simulink model "filter_2nd_order_iir_cosim"  (Simulink 6.4)
settings: Solver=FixedStepDiscrete  SolverMode=SingleTasking  StartTime=0.0  StopTime=0.1  RelTol=1e-3
undefined symbols (not defined in the file or in its folder): pipeline_prec
libraries: modelsimlib x1
settings Model: LastModifiedBy=Administrador

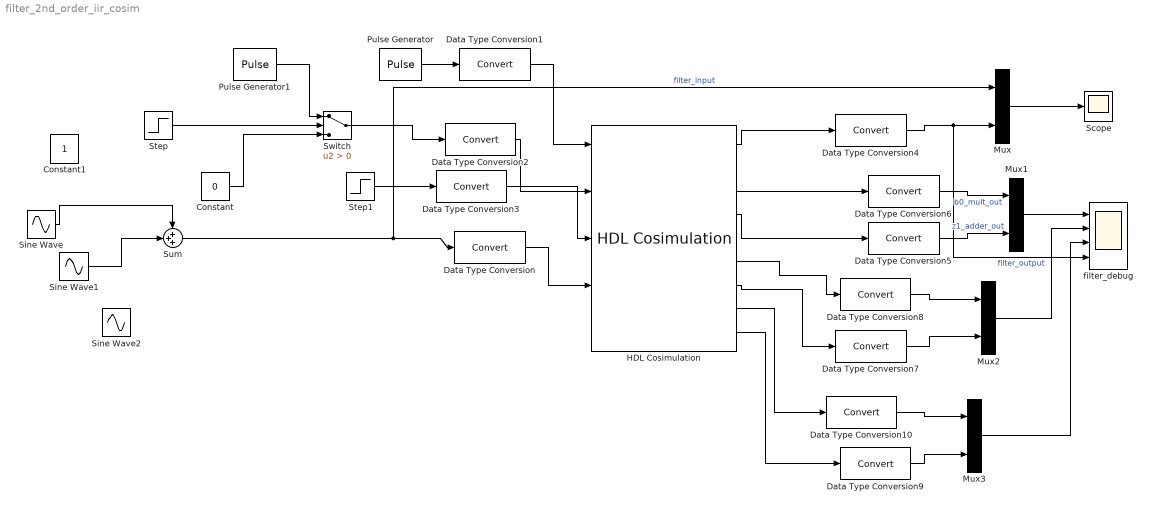
== system filter_2nd_order_iir_cosim ==
  Constant : Constant  Value=0  OutDataType=sfix(16)  ConRadixGroup=Use specified scaling  OutScaling=2^0  SampleTime=-1  FramePeriod=inf
  Constant1 : Constant  Value=1  OutDataType=sfix(16)  ConRadixGroup=Use specified scaling  OutScaling=2^0  SampleTime=-1  FramePeriod=inf
  Data Type Conversion : DataTypeConversion  OutDataTypeMode=Specify via dialog  OutDataType=sfix(18)  OutScaling=2^(-pipeline_prec)  RndMeth=Nearest  SampleTime=1e-5  SaturateOnIntegerOverflow=on
  Data Type Conversion1 : DataTypeConversion  OutDataTypeMode=boolean
  Data Type Conversion{4..10} (7 alike) : DataTypeConversion
  Data Type Conversion2 : DataTypeConversion  OutDataTypeMode=boolean
  Data Type Conversion3 : DataTypeConversion  OutDataTypeMode=boolean  SampleTime=0.5e-6
  HDL Cosimulation : modelsimlib/HDL Cosimulation  DialogController=modelsimddg.CoSim  DialogControllerArgs=DataTag0  PortPaths=/filter_2nd_order_iir_cosim_tb/iir_i/clk;/filter_2nd_order_iir_cosim_tb/iir_i/run_en;/filter_2nd_order_iir_cosim_tb/iir_i/rst;/filter_2nd_order_iir_cosim_tb/iir_i/i;/filter_2nd_order_iir_cosim_tb/iir_i/o;/filter_2nd_order_iir_cosim_tb/iir_i/run_passthru;/filter_2nd_order_iir_cosim_tb/iir_i/z1_adder_out_s;/filter_2nd_order_iir_cosim_tb/iir_i/z2_adder_out_s;/filter_2nd_order_iir_cosim_tb/iir_i/delayer_in;/filter_2nd_order_iir_cosim_tb/iir_i/delayer_out;/filter_2nd_order_iir_cosim_tb/iir_i/b1_mult_out_s;/filter_2nd_order_iir_cosim_tb/iir_i/a1_mult_out_s;/filter_2nd_order_iir_cosim_tb/iir_i/b2_mult_out_s;/filter_2nd_order_iir_cosim_tb/iir_i/a2_mult_out_s  PortModes=[1 1 1 1 2 2 2 2 1 2 2 2 2 2 ]  PortTimes=[1,1,1,1,1e-4,1,1e-4,1e-4,1,1,1e-4,1e-4,1e-4,1e-4]  PortSigns=[-1 -1 -1 -1 1 -1 1 1 -1 -1 1 1 1 1 ]  PortFracLengths=[0,0,0,0,pipeline_prec,0,pipeline_prec,pipeline_prec,0,0,pipeline_prec,pipeline_prec,pipeline_prec,pipeline_prec]  CommLocal=on  CommSharedMemory=off  CommPortNumber=4449  CommShowInfo=on  ClockModes=[]  ClockTimes=[]  TclPreSimCommand="echo \"Running Simulink Cosimulation block.\""  TclPostSimCommand="echo \"done\""  TimingMode=s  TimingScaleFactor=1  idxCellArray={'UNUSED_VAR'}
  Mux{,1..3} (4 alike) : Mux  Inputs=2
  Pulse Generator : DiscretePulseGenerator  PulseType=Time based  Period=1/(1e6)  PulseWidth=50
  Pulse Generator1 : DiscretePulseGenerator  PulseType=Time based  Period=0.1e-3  PulseWidth=0.5  PhaseDelay=4*(1/1e6)
  Scope : Scope
      settings: TimeRange=0.01  YMin=-1.75  YMax=1  MaxDataPoints=500000  Decimation=30
  Sine Wave : Sin  Frequency=2*pi*30  SampleTime=0
  Sine Wave1 : Sin  Frequency=2*pi*100  SampleTime=0
  Sine Wave2 : Sin  Frequency=100*2*pi  SampleTime=0
  Step : Step  Time=4*(1/1e6)
  Step1 : Step  Time=4e-6  Before=1  After=0
  Sum : Sum  Inputs=+++
  Switch : Switch  Criteria=u2 > Threshold  RndMeth=Nearest  ZeroCross=off  SampleTime=1e-7
  filter_debug : Scope  NumInputPorts=4
      settings: TimeRange=0.01  YMin=-2~-3.5~-5~-5  YMax=1.75~3.5~5~5  MaxDataPoints=500000
  wires:
  Pulse Generator/1 -> Data Type Conversion1/1
  Data Type Conversion1/1 -> HDL Cosimulation/1
  Switch/1 -> Data Type Conversion2/1
  Data Type Conversion2/1 -> HDL Cosimulation/2
  Step1/1 -> Data Type Conversion3/1
  Constant/1 -> Switch/3
  Step/1 -> Switch/2
  Pulse Generator1/1 -> Switch/1
  Data Type Conversion4/1 -> Mux/2, filter_debug/4  "filter_output"
  Sum/1 -> Data Type Conversion/1, Mux/1  "filter_input"
  Data Type Conversion3/1 -> HDL Cosimulation/3
  Data Type Conversion/1 -> HDL Cosimulation/4
  HDL Cosimulation/1 -> Data Type Conversion4/1
  HDL Cosimulation/4 -> Data Type Conversion5/1
  HDL Cosimulation/3 -> Data Type Conversion6/1
  Mux/1 -> Scope/1
  Sine Wave1/1 -> Sum/2
  Sine Wave/1 -> Sum/1
  Data Type Conversion6/1 -> Mux1/1  "b0_mult_out"
  Data Type Conversion5/1 -> Mux1/2  "z1_adder_out"
  Mux1/1 -> filter_debug/1
  Data Type Conversion8/1 -> Mux2/1
  Data Type Conversion7/1 -> Mux2/2
  Mux2/1 -> filter_debug/2
  HDL Cosimulation/6 -> Data Type Conversion8/1
  HDL Cosimulation/7 -> Data Type Conversion7/1
  Mux3/1 -> filter_debug/3
  Data Type Conversion10/1 -> Mux3/1
  Data Type Conversion9/1 -> Mux3/2
  HDL Cosimulation/8 -> Data Type Conversion10/1
  HDL Cosimulation/9 -> Data Type Conversion9/1
